simulink model "poco_ref_al_r307"  (Simulink 6.2)
settings: Solver=ode45  StartTime=0.0  StopTime=100000  RelTol=1e-3
libraries: xbsIndex_r3 x1012, xps_library x42, ddc_library x4, adcscope_lib x2, fft_library x2, pfb_library x2, delay_lib x1
(part 3 of 9)

== system poco_ref_al_r307/downshift2 ==
  din : Inport  Port=1  LatchInput=off
  Concat : xbsIndex_r3/Concat  num_inputs=2  explicit_period=off  period=1  dbl_ovrd=off
  Convert1 : xbsIndex_r3/Convert  arith_type="Signed  (2's comp)"  n_bits=18  bin_pt=15  quantization="Round  (unbiased: Even Values)"  overflow=Wrap  latency=2  explicit_period=off  period=1  dbl_ovrd=off  show_param=off  inserted_by_tool=off  pipeline=off
      settings: xl_area=[0, 0, 0, 0, 0, 0, 0]
  Convert2 : xbsIndex_r3/Convert  arith_type="Signed  (2's comp)"  n_bits=18  bin_pt=15  quantization="Round  (unbiased: Even Values)"  overflow=Wrap  latency=2  explicit_period=off  period=1  dbl_ovrd=off  show_param=off  inserted_by_tool=off  pipeline=off
      settings: xl_area=[0, 0, 0, 0, 0, 0, 0]
  Reinterpret : xbsIndex_r3/Reinterpret  force_arith_type=on  arith_type="Signed  (2's comp)"  force_bin_pt=on  bin_pt=17  force_valid=on
  Reinterpret1 : xbsIndex_r3/Reinterpret  force_arith_type=on  arith_type="Signed  (2's comp)"  force_bin_pt=on  bin_pt=17  force_valid=on
  Reinterpret3 : xbsIndex_r3/Reinterpret  force_arith_type=on  arith_type=Unsigned  force_bin_pt=on  bin_pt=0  force_valid=on
  Reinterpret4 : xbsIndex_r3/Reinterpret  force_arith_type=on  arith_type=Unsigned  force_bin_pt=on  bin_pt=0  force_valid=on
  Slice2 : xbsIndex_r3/Slice  mode=Upper Bit Location + Width  nbits=18  bit1=0  base1=MSB of Input  bit0=0  base0=LSB of Input  boolean_output=off  explicit_period=off  period=1  dbl_ovrd=off
  Slice20 : xbsIndex_r3/Slice  mode=Lower Bit Location + Width  nbits=18  bit1=0  base1=MSB of Input  bit0=0  base0=LSB of Input  boolean_output=off  explicit_period=off  period=1  dbl_ovrd=off
  dout : Outport
  wires:
  Convert1/1 -> Reinterpret4/1
  Convert2/1 -> Reinterpret3/1
  Reinterpret1/1 -> Convert1/1
  Reinterpret/1 -> Convert2/1
  Concat/1 -> dout/1
  Reinterpret4/1 -> Concat/2
  Reinterpret3/1 -> Concat/1
  din/1 -> Slice20/1, Slice2/1
  Slice20/1 -> Reinterpret1/1
  Slice2/1 -> Reinterpret/1

== system poco_ref_al_r307/downshift3 ==
  din : Inport  Port=1  LatchInput=off
  Concat : xbsIndex_r3/Concat  num_inputs=2  explicit_period=off  period=1  dbl_ovrd=off
  Convert1 : xbsIndex_r3/Convert  arith_type="Signed  (2's comp)"  n_bits=18  bin_pt=15  quantization="Round  (unbiased: Even Values)"  overflow=Wrap  latency=2  explicit_period=off  period=1  dbl_ovrd=off  show_param=off  inserted_by_tool=off  pipeline=off
      settings: xl_area=[0, 0, 0, 0, 0, 0, 0]
  Convert2 : xbsIndex_r3/Convert  arith_type="Signed  (2's comp)"  n_bits=18  bin_pt=15  quantization="Round  (unbiased: Even Values)"  overflow=Wrap  latency=2  explicit_period=off  period=1  dbl_ovrd=off  show_param=off  inserted_by_tool=off  pipeline=off
      settings: xl_area=[0, 0, 0, 0, 0, 0, 0]
  Reinterpret : xbsIndex_r3/Reinterpret  force_arith_type=on  arith_type="Signed  (2's comp)"  force_bin_pt=on  bin_pt=17  force_valid=on
  Reinterpret1 : xbsIndex_r3/Reinterpret  force_arith_type=on  arith_type="Signed  (2's comp)"  force_bin_pt=on  bin_pt=17  force_valid=on
  Reinterpret3 : xbsIndex_r3/Reinterpret  force_arith_type=on  arith_type=Unsigned  force_bin_pt=on  bin_pt=0  force_valid=on
  Reinterpret4 : xbsIndex_r3/Reinterpret  force_arith_type=on  arith_type=Unsigned  force_bin_pt=on  bin_pt=0  force_valid=on
  Slice2 : xbsIndex_r3/Slice  mode=Upper Bit Location + Width  nbits=18  bit1=0  base1=MSB of Input  bit0=0  base0=LSB of Input  boolean_output=off  explicit_period=off  period=1  dbl_ovrd=off
  Slice20 : xbsIndex_r3/Slice  mode=Lower Bit Location + Width  nbits=18  bit1=0  base1=MSB of Input  bit0=0  base0=LSB of Input  boolean_output=off  explicit_period=off  period=1  dbl_ovrd=off
  dout : Outport
  wires:
  Slice2/1 -> Reinterpret/1
  Slice20/1 -> Reinterpret1/1
  din/1 -> Slice2/1, Slice20/1
  Reinterpret3/1 -> Concat/1
  Reinterpret4/1 -> Concat/2
  Concat/1 -> dout/1
  Reinterpret/1 -> Convert2/1
  Reinterpret1/1 -> Convert1/1
  Convert2/1 -> Reinterpret3/1
  Convert1/1 -> Reinterpret4/1

== system poco_ref_al_r307/eq_ant0 ==
  sync : Inport  Port=1  LatchInput=off
  pol1 : Inport  Port=2  LatchInput=off
  pol2 : Inport  Port=3  LatchInput=off
  scale_pol1 : Inport  Port=4  LatchInput=off
  scale_pol2 : Inport  Port=5  LatchInput=off
  Concat3 : xbsIndex_r3/Concat  num_inputs=2  explicit_period=off  period=1  dbl_ovrd=off
  Delay1 : xbsIndex_r3/Delay  latency=1  reg_retiming=off  explicit_period=off  period=1  en=off  accept_only_valid=off  init_zero=on  dbl_ovrd=off  show_param=off
      settings: xl_area=[0, 0, 0, 0, 0, 0, 0]
  Delay11 : xbsIndex_r3/Delay  latency=1  reg_retiming=off  explicit_period=off  period=1  en=off  accept_only_valid=off  init_zero=on  dbl_ovrd=off  show_param=off
      settings: xl_area=[0, 0, 0, 0, 0, 0, 0]
  Delay4 : xbsIndex_r3/Delay  latency=5  reg_retiming=off  explicit_period=off  period=1  en=off  accept_only_valid=off  init_zero=on  dbl_ovrd=off  show_param=off
      settings: xl_area=[0, 0, 0, 0, 0, 0, 0]
  Logical1 : xbsIndex_r3/Logical  logical_function=OR  inputs=2  precision=Full  arith_type=Unsigned  n_bits=8  bin_pt=2  align_bp=on  latency=1  explicit_period=off  period=1  en=off  dbl_ovrd=off  show_param=off
      settings: xl_area=[0, 0, 0, 0, 0, 0, 0]
  round1 : Subsystem
  round2 : Subsystem
  dout : Outport
  sync_out : Outport  Port=2
  clip : Outport  Port=3
  wires:
  sync/1 -> Delay4/1
  round1/1(dout) -> Concat3/1
  round2/1(dout) -> Concat3/2
  Delay11/1 -> round1/1(din)
  Delay1/1 -> round2/1(din)
  pol1/1 -> Delay11/1
  pol2/1 -> Delay1/1
  Concat3/1 -> dout/1
  Delay4/1 -> sync_out/1
  round1/2(clip) -> Logical1/1
  round2/2(clip) -> Logical1/2
  Logical1/1 -> clip/1
  scale_pol1/1 -> round1/2(scale)
  scale_pol2/1 -> round2/2(scale)

== system poco_ref_al_r307/eq_ant1 ==
  sync : Inport  Port=1  LatchInput=off
  pol1 : Inport  Port=2  LatchInput=off
  pol2 : Inport  Port=3  LatchInput=off
  scale_pol1 : Inport  Port=4  LatchInput=off
  scale_pol2 : Inport  Port=5  LatchInput=off
  Concat3 : xbsIndex_r3/Concat  num_inputs=2  explicit_period=off  period=1  dbl_ovrd=off
  Delay1 : xbsIndex_r3/Delay  latency=1  reg_retiming=off  explicit_period=off  period=1  en=off  accept_only_valid=off  init_zero=on  dbl_ovrd=off  show_param=off
      settings: xl_area=[0, 0, 0, 0, 0, 0, 0]
  Delay11 : xbsIndex_r3/Delay  latency=1  reg_retiming=off  explicit_period=off  period=1  en=off  accept_only_valid=off  init_zero=on  dbl_ovrd=off  show_param=off
      settings: xl_area=[0, 0, 0, 0, 0, 0, 0]
  Delay4 : xbsIndex_r3/Delay  latency=5  reg_retiming=off  explicit_period=off  period=1  en=off  accept_only_valid=off  init_zero=on  dbl_ovrd=off  show_param=off
      settings: xl_area=[0, 0, 0, 0, 0, 0, 0]
  Logical1 : xbsIndex_r3/Logical  logical_function=OR  inputs=2  precision=Full  arith_type=Unsigned  n_bits=8  bin_pt=2  align_bp=on  latency=1  explicit_period=off  period=1  en=off  dbl_ovrd=off  show_param=off
      settings: xl_area=[0, 0, 0, 0, 0, 0, 0]
  round1 : Subsystem
  round2 : Subsystem
  dout : Outport
  sync_out : Outport  Port=2
  clip : Outport  Port=3
  wires:
  scale_pol2/1 -> round2/2(scale)
  scale_pol1/1 -> round1/2(scale)
  Logical1/1 -> clip/1
  round2/2(clip) -> Logical1/2
  round1/2(clip) -> Logical1/1
  Delay4/1 -> sync_out/1
  Concat3/1 -> dout/1
  pol2/1 -> Delay1/1
  pol1/1 -> Delay11/1
  Delay1/1 -> round2/1(din)
  Delay11/1 -> round1/1(din)
  round2/1(dout) -> Concat3/2
  round1/1(dout) -> Concat3/1
  sync/1 -> Delay4/1

== system poco_ref_al_r307/eq_prog ==
  sync : Inport  Port=1  LatchInput=off
  data_in : Inport  Port=2  LatchInput=off
  addr_in : Inport  Port=3  LatchInput=off
  valid_in : Inport  Port=4  LatchInput=off
  Constant : xbsIndex_r3/Constant  const=addr_offset  equ=P=C  arith_type=Unsigned  n_bits=32-addr_width  bin_pt=0  opselect=C  inp2=PCIN>>17  opr=+  inp1=P  carry=CIN  iostate=0  explicit_period=on  period=1  dbl_ovrd=off
  Constant5 : xbsIndex_r3/Constant  const=0  equ=P=C  arith_type=Unsigned  n_bits=16  bin_pt=3  opselect=C  inp2=PCIN>>17  opr=+  inp1=P  carry=CIN  iostate=0  explicit_period=on  period=1  dbl_ovrd=off
  Constant6 : xbsIndex_r3/Constant  const=0  equ=P=C  arith_type=Boolean  n_bits=1  bin_pt=0  opselect=C  inp2=PCIN>>17  opr=+  inp1=P  carry=CIN  iostate=0  explicit_period=on  period=1  dbl_ovrd=off
  Counter2 : xbsIndex_r3/Counter  cnt_type=Free Running  n_bits=chan_bits  bin_pt=0  arith_type=Unsigned  start_count=0  cnt_to=Inf  cnt_by_val=1  operation=Up  explicit_period=off  period=1  load_pin=off  rst=on  en=off  dbl_ovrd=off  show_param=off  use_rpm=on  gen_core=off
      settings: xl_area=[0, 0, 0, 0, 0, 0, 0]
  Dual Port RAM : xbsIndex_r3/Dual Port RAM  depth=n_chans  initVector=ones(1,n_chans)*1000  write_mode_A=Read After Write  write_mode_B=Read After Write  latency=1  mem_collision=off  init_zero=on  explicit_period=off  period=1  dbl_ovrd=off  rst_a=off  init_a=0  rst_b=off  init_b=0  show_param=off  distributed_mem=off  use_rpm=off  gen_core=off
      settings: xl_area=[0, 0, 0, 0, 0, 0, 0]
  Logical : xbsIndex_r3/Logical  logical_function=AND  inputs=2  precision=Full  arith_type=Unsigned  n_bits=8  bin_pt=2  align_bp=on  latency=0  explicit_period=off  period=1  en=off  dbl_ovrd=off  show_param=off
      settings: xl_area=[0, 0, 0, 0, 0, 0, 0]
  Register1 : xbsIndex_r3/Register  init=0  reg_only_valid=off  explicit_period=on  period=1  rst=off  en=off  out_en=off  dbl_ovrd=off  show_param=off
      settings: xl_area=[0, 0, 0, 0, 0, 0, 0]
  Register2 : xbsIndex_r3/Register  init=0  reg_only_valid=off  explicit_period=on  period=1  rst=off  en=off  out_en=off  dbl_ovrd=off  show_param=off
      settings: xl_area=[0, 0, 0, 0, 0, 0, 0]
  Register3 : xbsIndex_r3/Register  init=0  reg_only_valid=off  explicit_period=on  period=1  rst=off  en=off  out_en=off  dbl_ovrd=off  show_param=off
      settings: xl_area=[0, 0, 0, 0, 0, 0, 0]
  Reinterpret1 : xbsIndex_r3/Reinterpret  force_arith_type=on  arith_type=Unsigned  force_bin_pt=on  bin_pt=3  force_valid=on
  Relational : xbsIndex_r3/Relational  mode=a=b  latency=1  explicit_period=on  period=1  en=off  dbl_ovrd=off  show_param=off
      settings: xl_area=[0, 0, 0, 0, 0, 0, 0]
  Slice22 : xbsIndex_r3/Slice  mode=Lower Bit Location + Width  nbits=32-addr_width  bit1=0  base1=MSB of Input  bit0=addr_width  base0=LSB of Input  boolean_output=off  explicit_period=off  period=1  dbl_ovrd=off
  Slice9 : xbsIndex_r3/Slice  mode=Lower Bit Location + Width  nbits=addr_width  bit1=0  base1=MSB of Input  bit0=0  base0=LSB of Input  boolean_output=off  explicit_period=off  period=1  dbl_ovrd=off
  scale : Outport
  wires:
  addr_in/1 -> Slice9/1, Slice22/1
  Slice22/1 -> Relational/1
  Constant/1 -> Relational/2
  Relational/1 -> Logical/1
  valid_in/1 -> Register3/1
  Logical/1 -> Dual Port RAM/6
  Slice9/1 -> Register2/1
  data_in/1 -> Register1/1
  Register1/1 -> Reinterpret1/1
  Register2/1 -> Dual Port RAM/4
  Register3/1 -> Logical/2
  Counter2/1 -> Dual Port RAM/1
  Constant5/1 -> Dual Port RAM/2
  Constant6/1 -> Dual Port RAM/3
  Reinterpret1/1 -> Dual Port RAM/5
  sync/1 -> Counter2/1
  Dual Port RAM/1 -> scale/1

== system poco_ref_al_r307/pulse_ext1 ==
  in : Inport  Port=1  LatchInput=off
  Constant5 : xbsIndex_r3/Constant  const=pulse_len  equ=P=C  arith_type=Unsigned  n_bits=bits  bin_pt=0  opselect=C  inp2=PCIN>>17  opr=+  inp1=P  carry=CIN  iostate=0  explicit_period=off  period=1  dbl_ovrd=off
  Counter3 : xbsIndex_r3/Counter  cnt_type=Free Running  n_bits=bits  bin_pt=0  arith_type=Unsigned  start_count=0  cnt_to=1023  cnt_by_val=1  operation=Up  explicit_period=on  period=1  load_pin=off  rst=on  en=on  dbl_ovrd=off  show_param=off  use_rpm=on  gen_core=off
      settings: xl_area=[0, 0, 0, 0, 0, 0, 0]
  Relational5 : xbsIndex_r3/Relational  mode=a!=b  latency=0  explicit_period=off  period=1  en=off  dbl_ovrd=off  show_param=off
      settings: xl_area=[0, 0, 0, 0, 0, 0, 0]
  posedge : Subsystem  Tag=Rising Edge Detector
  out : Outport
  wires:
  posedge/1(Out) -> Counter3/1
  in/1 -> posedge/1(In)
  Relational5/1 -> out/1, Counter3/2
  Constant5/1 -> Relational5/2
  Counter3/1 -> Relational5/1

== system poco_ref_al_r307/pulse_ext2 ==
  in : Inport  Port=1  LatchInput=off
  Constant5 : xbsIndex_r3/Constant  const=pulse_len  equ=P=C  arith_type=Unsigned  n_bits=bits  bin_pt=0  opselect=C  inp2=PCIN>>17  opr=+  inp1=P  carry=CIN  iostate=0  explicit_period=off  period=1  dbl_ovrd=off
  Counter3 : xbsIndex_r3/Counter  cnt_type=Free Running  n_bits=bits  bin_pt=0  arith_type=Unsigned  start_count=0  cnt_to=1023  cnt_by_val=1  operation=Up  explicit_period=on  period=1  load_pin=off  rst=on  en=on  dbl_ovrd=off  show_param=off  use_rpm=on  gen_core=off
      settings: xl_area=[0, 0, 0, 0, 0, 0, 0]
  Relational5 : xbsIndex_r3/Relational  mode=a!=b  latency=0  explicit_period=off  period=1  en=off  dbl_ovrd=off  show_param=off
      settings: xl_area=[0, 0, 0, 0, 0, 0, 0]
  posedge : Subsystem  Tag=Rising Edge Detector
  out : Outport
  wires:
  Counter3/1 -> Relational5/1
  Constant5/1 -> Relational5/2
  Relational5/1 -> Counter3/2, out/1
  in/1 -> posedge/1(In)
  posedge/1(Out) -> Counter3/1

== system poco_ref_al_r307/pulse_ext3 ==
  in : Inport  Port=1  LatchInput=off
  Constant5 : xbsIndex_r3/Constant  const=pulse_len  equ=P=C  arith_type=Unsigned  n_bits=bits  bin_pt=0  opselect=C  inp2=PCIN>>17  opr=+  inp1=P  carry=CIN  iostate=0  explicit_period=off  period=1  dbl_ovrd=off
  Counter3 : xbsIndex_r3/Counter  cnt_type=Free Running  n_bits=bits  bin_pt=0  arith_type=Unsigned  start_count=0  cnt_to=1023  cnt_by_val=1  operation=Up  explicit_period=on  period=1  load_pin=off  rst=on  en=on  dbl_ovrd=off  show_param=off  use_rpm=on  gen_core=off
      settings: xl_area=[0, 0, 0, 0, 0, 0, 0]
  Relational5 : xbsIndex_r3/Relational  mode=a!=b  latency=0  explicit_period=off  period=1  en=off  dbl_ovrd=off  show_param=off
      settings: xl_area=[0, 0, 0, 0, 0, 0, 0]
  posedge : Subsystem  Tag=Rising Edge Detector
  out : Outport
  wires:
  Counter3/1 -> Relational5/1
  Constant5/1 -> Relational5/2
  Relational5/1 -> Counter3/2, out/1
  in/1 -> posedge/1(In)
  posedge/1(Out) -> Counter3/1

== system poco_ref_al_r307/pulse_ext4 ==
  in : Inport  Port=1  LatchInput=off
  Constant5 : xbsIndex_r3/Constant  const=pulse_len  equ=P=C  arith_type=Unsigned  n_bits=bits  bin_pt=0  opselect=C  inp2=PCIN>>17  opr=+  inp1=P  carry=CIN  iostate=0  explicit_period=off  period=1  dbl_ovrd=off
  Counter3 : xbsIndex_r3/Counter  cnt_type=Free Running  n_bits=bits  bin_pt=0  arith_type=Unsigned  start_count=0  cnt_to=1023  cnt_by_val=1  operation=Up  explicit_period=on  period=1  load_pin=off  rst=on  en=on  dbl_ovrd=off  show_param=off  use_rpm=on  gen_core=off
      settings: xl_area=[0, 0, 0, 0, 0, 0, 0]
  Relational5 : xbsIndex_r3/Relational  mode=a!=b  latency=0  explicit_period=off  period=1  en=off  dbl_ovrd=off  show_param=off
      settings: xl_area=[0, 0, 0, 0, 0, 0, 0]
  posedge : Subsystem  Tag=Rising Edge Detector
  out : Outport
  wires:
  Counter3/1 -> Relational5/1
  Constant5/1 -> Relational5/2
  Relational5/1 -> Counter3/2, out/1
  in/1 -> posedge/1(In)
  posedge/1(Out) -> Counter3/1

== system poco_ref_al_r307/pulse_ext5 ==
  in : Inport  Port=1  LatchInput=off
  Constant5 : xbsIndex_r3/Constant  const=pulse_len  equ=P=C  arith_type=Unsigned  n_bits=bits  bin_pt=0  opselect=C  inp2=PCIN>>17  opr=+  inp1=P  carry=CIN  iostate=0  explicit_period=off  period=1  dbl_ovrd=off
  Counter3 : xbsIndex_r3/Counter  cnt_type=Free Running  n_bits=bits  bin_pt=0  arith_type=Unsigned  start_count=0  cnt_to=1023  cnt_by_val=1  operation=Up  explicit_period=on  period=1  load_pin=off  rst=on  en=on  dbl_ovrd=off  show_param=off  use_rpm=on  gen_core=off
      settings: xl_area=[0, 0, 0, 0, 0, 0, 0]
  Relational5 : xbsIndex_r3/Relational  mode=a!=b  latency=0  explicit_period=off  period=1  en=off  dbl_ovrd=off  show_param=off
      settings: xl_area=[0, 0, 0, 0, 0, 0, 0]
  posedge : Subsystem  Tag=Rising Edge Detector
  out : Outport
  wires:
  posedge/1(Out) -> Counter3/1
  in/1 -> posedge/1(In)
  Relational5/1 -> out/1, Counter3/2
  Constant5/1 -> Relational5/2
  Counter3/1 -> Relational5/1

== system poco_ref_al_r307/pulse_ext6 ==
  in : Inport  Port=1  LatchInput=off
  Constant5 : xbsIndex_r3/Constant  const=pulse_len  equ=P=C  arith_type=Unsigned  n_bits=bits  bin_pt=0  opselect=C  inp2=PCIN>>17  opr=+  inp1=P  carry=CIN  iostate=0  explicit_period=off  period=1  dbl_ovrd=off
  Counter3 : xbsIndex_r3/Counter  cnt_type=Free Running  n_bits=bits  bin_pt=0  arith_type=Unsigned  start_count=0  cnt_to=1023  cnt_by_val=1  operation=Up  explicit_period=on  period=1  load_pin=off  rst=on  en=on  dbl_ovrd=off  show_param=off  use_rpm=on  gen_core=off
      settings: xl_area=[0, 0, 0, 0, 0, 0, 0]
  Relational5 : xbsIndex_r3/Relational  mode=a!=b  latency=0  explicit_period=off  period=1  en=off  dbl_ovrd=off  show_param=off
      settings: xl_area=[0, 0, 0, 0, 0, 0, 0]
  posedge : Subsystem  Tag=Rising Edge Detector
  out : Outport
  wires:
  posedge/1(Out) -> Counter3/1
  in/1 -> posedge/1(In)
  Relational5/1 -> out/1, Counter3/2
  Constant5/1 -> Relational5/2
  Counter3/1 -> Relational5/1

== system poco_ref_al_r307/pulse_ext7 ==
  in : Inport  Port=1  LatchInput=off
  Constant5 : xbsIndex_r3/Constant  const=pulse_len  equ=P=C  arith_type=Unsigned  n_bits=bits  bin_pt=0  opselect=C  inp2=PCIN>>17  opr=+  inp1=P  carry=CIN  iostate=0  explicit_period=off  period=1  dbl_ovrd=off
  Counter3 : xbsIndex_r3/Counter  cnt_type=Free Running  n_bits=bits  bin_pt=0  arith_type=Unsigned  start_count=0  cnt_to=1023  cnt_by_val=1  operation=Up  explicit_period=on  period=1  load_pin=off  rst=on  en=on  dbl_ovrd=off  show_param=off  use_rpm=on  gen_core=off
      settings: xl_area=[0, 0, 0, 0, 0, 0, 0]
  Relational5 : xbsIndex_r3/Relational  mode=a!=b  latency=0  explicit_period=off  period=1  en=off  dbl_ovrd=off  show_param=off
      settings: xl_area=[0, 0, 0, 0, 0, 0, 0]
  posedge : Subsystem  Tag=Rising Edge Detector
  out : Outport
  wires:
  posedge/1(Out) -> Counter3/1
  in/1 -> posedge/1(In)
  Relational5/1 -> out/1, Counter3/2
  Constant5/1 -> Relational5/2
  Counter3/1 -> Relational5/1

== system poco_ref_al_r307/sync_gen ==
  note: sync_delay makes sure mrst
      | gets transmitted
      | on a correctly aligned sync
  rst : Inport  Port=1  LatchInput=off
  arm : Inport  Port=2  LatchInput=off
  Constant10 : xbsIndex_r3/Constant  const=1  equ=P=C  arith_type=Boolean  n_bits=1  bin_pt=0  opselect=C  inp2=PCIN>>17  opr=+  inp1=P  carry=CIN  iostate=0  explicit_period=on  period=1  dbl_ovrd=off
  Counter : xbsIndex_r3/Counter  cnt_type=Free Running  n_bits=sync_bits+1  bin_pt=0  arith_type=Unsigned  start_count=0  cnt_to=Inf  cnt_by_val=1  operation=Up  explicit_period=off  period=1  load_pin=off  rst=on  en=off  dbl_ovrd=off  show_param=off  use_rpm=on  gen_core=off
      settings: xl_area=[0, 0, 0, 0, 0, 0, 0]
  Inverter : xbsIndex_r3/Inverter  latency=2  explicit_period=off  period=1  en=off  dbl_ovrd=off  show_param=off
      settings: xl_area=[0, 0, 0, 0, 0, 0, 0]
  Register : xbsIndex_r3/Register  init=0  reg_only_valid=off  explicit_period=off  period=1  rst=on  en=on  out_en=off  dbl_ovrd=off  show_param=off
      settings: xl_area=[0, 0, 0, 0, 0, 0, 0]
  Slice8 : xbsIndex_r3/Slice  mode=Upper Bit Location + Width  nbits=1  bit1=0  base1=MSB of Input  bit0=19  base0=LSB of Input  boolean_output=on  explicit_period=off  period=1  dbl_ovrd=off
  edge : Subsystem
  posedge1 : Subsystem  Tag=Rising Edge Detector
  posedge2 : Subsystem  Tag=Rising Edge Detector
  sync_delay : delay_lib/sync_delay  DelayLen=2^sync_bits
      link override Constant: equ=P=C
      link override Constant1: equ=P=C
      link override Constant2: equ=P=C
      link override Constant3: equ=P=C
  sync : Outport
  mrst : Outport  Port=2
  armed : Outport  Port=3
  wires:
  Counter/1 -> Slice8/1
  posedge1/1(Out) -> Counter/1, sync_delay/1
  Register/1 -> posedge1/1(In), Inverter/1
  Constant10/1 -> Register/1
  posedge2/1(Out) -> Register/2
  arm/1 -> posedge2/1(In)
  rst/1 -> Register/3
  sync_delay/1 -> mrst/1
  Slice8/1 -> edge/1(in)
  edge/1(out) -> sync/1
  Inverter/1 -> armed/1

== system poco_ref_al_r307/acc_cntrl/posedge1 ==
  In : Inport  Port=1  LatchInput=off
  Delay : xbsIndex_r3/Delay  latency=1  reg_retiming=off  explicit_period=off  period=1  en=off  accept_only_valid=off  init_zero=on  dbl_ovrd=off  show_param=off
      settings: xl_area=[0, 0, 0, 0, 0, 0, 0]
  Inverter : xbsIndex_r3/Inverter  latency=0  explicit_period=off  period=1  en=off  dbl_ovrd=off  show_param=off
      settings: xl_area=[0, 0, 0, 0, 0, 0, 0]
  Logical : xbsIndex_r3/Logical  logical_function=AND  inputs=2  precision=Full  arith_type=Unsigned  n_bits=8  bin_pt=2  align_bp=on  latency=0  explicit_period=off  period=1  en=off  dbl_ovrd=off  show_param=off
      settings: xl_area=[0, 0, 0, 0, 0, 0, 0]
  Out : Outport
  wires:
  Logical/1 -> Out/1
  In/1 -> Logical/2, Delay/1
  Inverter/1 -> Logical/1
  Delay/1 -> Inverter/1

== system poco_ref_al_r307/acc_cntrl/posedge2 ==
  In : Inport  Port=1  LatchInput=off
  Delay : xbsIndex_r3/Delay  latency=1  reg_retiming=off  explicit_period=off  period=1  en=off  accept_only_valid=off  init_zero=on  dbl_ovrd=off  show_param=off
      settings: xl_area=[0, 0, 0, 0, 0, 0, 0]
  Inverter : xbsIndex_r3/Inverter  latency=0  explicit_period=off  period=1  en=off  dbl_ovrd=off  show_param=off
      settings: xl_area=[0, 0, 0, 0, 0, 0, 0]
  Logical : xbsIndex_r3/Logical  logical_function=AND  inputs=2  precision=Full  arith_type=Unsigned  n_bits=8  bin_pt=2  align_bp=on  latency=0  explicit_period=off  period=1  en=off  dbl_ovrd=off  show_param=off
      settings: xl_area=[0, 0, 0, 0, 0, 0, 0]
  Out : Outport
  wires:
  Delay/1 -> Inverter/1
  Inverter/1 -> Logical/1
  In/1 -> Delay/1, Logical/2
  Logical/1 -> Out/1

== system poco_ref_al_r307/calc_adc_sum_sq1/decat4 ==
  In1 : Inport  Port=1  LatchInput=off
  Reinterpret{1..4} (4 alike) : xbsIndex_r3/Reinterpret  force_arith_type=on  arith_type="Signed  (2's comp)"  force_bin_pt=on  bin_pt=7  force_valid=on
  Slice15 : xbsIndex_r3/Slice  mode=Lower Bit Location + Width  nbits=8  bit1=0  base1=MSB of Input  bit0=8  base0=LSB of Input  boolean_output=off  explicit_period=off  period=1  dbl_ovrd=off
  Slice16 : xbsIndex_r3/Slice  mode=Lower Bit Location + Width  nbits=8  bit1=0  base1=MSB of Input  bit0=16  base0=LSB of Input  boolean_output=off  explicit_period=off  period=1  dbl_ovrd=off
  Slice17 : xbsIndex_r3/Slice  mode=Lower Bit Location + Width  nbits=8  bit1=0  base1=MSB of Input  bit0=24  base0=LSB of Input  boolean_output=off  explicit_period=off  period=1  dbl_ovrd=off
  Slice9 : xbsIndex_r3/Slice  mode=Lower Bit Location + Width  nbits=8  bit1=0  base1=MSB of Input  bit0=0  base0=LSB of Input  boolean_output=off  explicit_period=off  period=1  dbl_ovrd=off
  Out1 : Outport
  Out2 : Outport  Port=2
  Out3 : Outport  Port=3
  Out4 : Outport  Port=4
  wires:
  Reinterpret4/1 -> Out4/1
  Reinterpret3/1 -> Out3/1
  Reinterpret1/1 -> Out2/1
  Reinterpret2/1 -> Out1/1
  Slice9/1 -> Reinterpret4/1
  Slice15/1 -> Reinterpret3/1
  Slice16/1 -> Reinterpret1/1
  Slice17/1 -> Reinterpret2/1
  In1/1 -> Slice15/1, Slice9/1, Slice16/1, Slice17/1

== system poco_ref_al_r307/calc_adc_sum_sq2/decat4 ==
  In1 : Inport  Port=1  LatchInput=off
  Reinterpret{1..4} (4 alike) : xbsIndex_r3/Reinterpret  force_arith_type=on  arith_type="Signed  (2's comp)"  force_bin_pt=on  bin_pt=7  force_valid=on
  Slice15 : xbsIndex_r3/Slice  mode=Lower Bit Location + Width  nbits=8  bit1=0  base1=MSB of Input  bit0=8  base0=LSB of Input  boolean_output=off  explicit_period=off  period=1  dbl_ovrd=off
  Slice16 : xbsIndex_r3/Slice  mode=Lower Bit Location + Width  nbits=8  bit1=0  base1=MSB of Input  bit0=16  base0=LSB of Input  boolean_output=off  explicit_period=off  period=1  dbl_ovrd=off
  Slice17 : xbsIndex_r3/Slice  mode=Lower Bit Location + Width  nbits=8  bit1=0  base1=MSB of Input  bit0=24  base0=LSB of Input  boolean_output=off  explicit_period=off  period=1  dbl_ovrd=off
  Slice9 : xbsIndex_r3/Slice  mode=Lower Bit Location + Width  nbits=8  bit1=0  base1=MSB of Input  bit0=0  base0=LSB of Input  boolean_output=off  explicit_period=off  period=1  dbl_ovrd=off
  Out1 : Outport
  Out2 : Outport  Port=2
  Out3 : Outport  Port=3
  Out4 : Outport  Port=4
  wires:
  Reinterpret4/1 -> Out4/1
  Reinterpret3/1 -> Out3/1
  Reinterpret1/1 -> Out2/1
  Reinterpret2/1 -> Out1/1
  Slice9/1 -> Reinterpret4/1
  Slice15/1 -> Reinterpret3/1
  Slice16/1 -> Reinterpret1/1
  Slice17/1 -> Reinterpret2/1
  In1/1 -> Slice15/1, Slice9/1, Slice16/1, Slice17/1

== system poco_ref_al_r307/calc_adc_sum_sq3/decat4 ==
  In1 : Inport  Port=1  LatchInput=off
  Reinterpret{1..4} (4 alike) : xbsIndex_r3/Reinterpret  force_arith_type=on  arith_type="Signed  (2's comp)"  force_bin_pt=on  bin_pt=7  force_valid=on
  Slice15 : xbsIndex_r3/Slice  mode=Lower Bit Location + Width  nbits=8  bit1=0  base1=MSB of Input  bit0=8  base0=LSB of Input  boolean_output=off  explicit_period=off  period=1  dbl_ovrd=off
  Slice16 : xbsIndex_r3/Slice  mode=Lower Bit Location + Width  nbits=8  bit1=0  base1=MSB of Input  bit0=16  base0=LSB of Input  boolean_output=off  explicit_period=off  period=1  dbl_ovrd=off
  Slice17 : xbsIndex_r3/Slice  mode=Lower Bit Location + Width  nbits=8  bit1=0  base1=MSB of Input  bit0=24  base0=LSB of Input  boolean_output=off  explicit_period=off  period=1  dbl_ovrd=off
  Slice9 : xbsIndex_r3/Slice  mode=Lower Bit Location + Width  nbits=8  bit1=0  base1=MSB of Input  bit0=0  base0=LSB of Input  boolean_output=off  explicit_period=off  period=1  dbl_ovrd=off
  Out1 : Outport
  Out2 : Outport  Port=2
  Out3 : Outport  Port=3
  Out4 : Outport  Port=4
  wires:
  Reinterpret4/1 -> Out4/1
  Reinterpret3/1 -> Out3/1
  Reinterpret1/1 -> Out2/1
  Reinterpret2/1 -> Out1/1
  Slice9/1 -> Reinterpret4/1
  Slice15/1 -> Reinterpret3/1
  Slice16/1 -> Reinterpret1/1
  Slice17/1 -> Reinterpret2/1
  In1/1 -> Slice15/1, Slice9/1, Slice16/1, Slice17/1

== system poco_ref_al_r307/calc_adc_sum_sq4/decat4 ==
  In1 : Inport  Port=1  LatchInput=off
  Reinterpret{1..4} (4 alike) : xbsIndex_r3/Reinterpret  force_arith_type=on  arith_type="Signed  (2's comp)"  force_bin_pt=on  bin_pt=7  force_valid=on
  Slice15 : xbsIndex_r3/Slice  mode=Lower Bit Location + Width  nbits=8  bit1=0  base1=MSB of Input  bit0=8  base0=LSB of Input  boolean_output=off  explicit_period=off  period=1  dbl_ovrd=off
  Slice16 : xbsIndex_r3/Slice  mode=Lower Bit Location + Width  nbits=8  bit1=0  base1=MSB of Input  bit0=16  base0=LSB of Input  boolean_output=off  explicit_period=off  period=1  dbl_ovrd=off
  Slice17 : xbsIndex_r3/Slice  mode=Lower Bit Location + Width  nbits=8  bit1=0  base1=MSB of Input  bit0=24  base0=LSB of Input  boolean_output=off  explicit_period=off  period=1  dbl_ovrd=off
  Slice9 : xbsIndex_r3/Slice  mode=Lower Bit Location + Width  nbits=8  bit1=0  base1=MSB of Input  bit0=0  base0=LSB of Input  boolean_output=off  explicit_period=off  period=1  dbl_ovrd=off
  Out1 : Outport
  Out2 : Outport  Port=2
  Out3 : Outport  Port=3
  Out4 : Outport  Port=4
  wires:
  Reinterpret4/1 -> Out4/1
  Reinterpret3/1 -> Out3/1
  Reinterpret1/1 -> Out2/1
  Reinterpret2/1 -> Out1/1
  Slice9/1 -> Reinterpret4/1
  Slice15/1 -> Reinterpret3/1
  Slice16/1 -> Reinterpret1/1
  Slice17/1 -> Reinterpret2/1
  In1/1 -> Slice15/1, Slice9/1, Slice16/1, Slice17/1

== system poco_ref_al_r307/delay_wideband_prog0/barrel_switcher ==
  sel : Inport  Port=1  LatchInput=off
  sync_in : Inport  Port=2  LatchInput=off
  In1 : Inport  Port=3  LatchInput=off
  In2 : Inport  Port=4  LatchInput=off
  In3 : Inport  Port=5  LatchInput=off
  In4 : Inport  Port=6  LatchInput=off
  Delay1 : xbsIndex_r3/Delay  latency=1  reg_retiming=off  explicit_period=off  period=1  en=off  accept_only_valid=off  init_zero=on  dbl_ovrd=off  show_param=off
      settings: xl_area=[0, 0, 0, 0, 0, 0, 0]
  Delay_sync : xbsIndex_r3/Delay  latency=2  reg_retiming=off  explicit_period=off  period=1  en=off  accept_only_valid=off  init_zero=on  dbl_ovrd=off  show_param=off
      settings: xl_area=[0, 0, 0, 0, 0, 0, 0]
  Mux{11..12,21..22,31..32,41..42} (8 alike) : xbsIndex_r3/Mux  inputs=2  precision=Full  arith_type="Signed  (2's comp)"  n_bits=8  bin_pt=2  quantization=Truncate  overflow=Wrap  latency=1  explicit_period=off  period=1  en=off  dbl_ovrd=off  show_param=off  mux_type=off  use_rpm=off  gen_core=off
      settings: xl_area=[0, 0, 0, 0, 0, 0, 0]
  Slice1 : xbsIndex_r3/Slice  mode=Upper Bit Location + Width  nbits=1  bit1=-0  base1=MSB of Input  bit0=0  base0=LSB of Input  boolean_output=off  explicit_period=off  period=1  dbl_ovrd=off
  Slice2 : xbsIndex_r3/Slice  mode=Upper Bit Location + Width  nbits=1  bit1=-1  base1=MSB of Input  bit0=0  base0=LSB of Input  boolean_output=off  explicit_period=off  period=1  dbl_ovrd=off
  sync_out : Outport
  Out1 : Outport  Port=2
  Out2 : Outport  Port=3
  Out3 : Outport  Port=4
  Out4 : Outport  Port=5
  wires:
  sync_in/1 -> Delay_sync/1
  Delay_sync/1 -> sync_out/1
  sel/1 -> Slice1/1, Delay1/1
  Delay1/1 -> Slice2/1
  Slice1/1 -> Mux11/1, Mux21/1, Mux31/1, Mux41/1
  Slice2/1 -> Mux12/1, Mux22/1, Mux32/1, Mux42/1
  In1/1 -> Mux11/2, Mux31/3
  Mux12/1 -> Out1/1
  In2/1 -> Mux21/2, Mux41/3
  Mux22/1 -> Out2/1
  In3/1 -> Mux31/2, Mux11/3
  Mux32/1 -> Out3/1
  In4/1 -> Mux41/2, Mux21/3
  Mux42/1 -> Out4/1
  Mux11/1 -> Mux12/2, Mux42/3
  Mux21/1 -> Mux22/2, Mux12/3
  Mux31/1 -> Mux32/2, Mux22/3
  Mux41/1 -> Mux42/2, Mux32/3

== system poco_ref_al_r307/delay_wideband_prog0/delay_dp ==
  din : Inport  Port=1  LatchInput=off
  delay : Inport  Port=2  LatchInput=off
  AddSub : xbsIndex_r3/AddSub  mode=Subtraction  precision=User Defined  arith_type=Unsigned  n_bits=11  bin_pt=0  quantization=Truncate  overflow=Wrap  latency=1  explicit_period=off  period=1  use_carryin=off  use_carryout=off  en=off  dbl_ovrd=off  show_param=off  use_core=on  pipeline=off  use_rpm=on  gen_core=off
      settings: xl_area=[0, 0, 0, 0, 0, 0, 0]
  Constant2 : xbsIndex_r3/Constant  const=1  equ=P=C  arith_type=Boolean  n_bits=1  bin_pt=0  opselect=C  inp2=PCIN>>17  opr=+  inp1=P  carry=CIN  iostate=0  explicit_period=on  period=1  dbl_ovrd=off
  Constant4 : xbsIndex_r3/Constant  const=0  equ=P=C  arith_type=Boolean  n_bits=1  bin_pt=0  opselect=C  inp2=PCIN>>17  opr=+  inp1=P  carry=CIN  iostate=0  explicit_period=on  period=1  dbl_ovrd=off
  Dual Port RAM : S-Function  AncestorBlock=xbsIndex_r3/Dual Port RAM  FunctionName=xldpram  Parameters=sfcn_mwsv__  mask(Xilinx Dual Port Random Access Memory){depth=2048, initVector=0, write_mode_A=Read After Write, write_mode_B=Read After Write, latency=4, mem_collision=off, init_zero=on, explicit_period=off, period=1, dbl_ovrd=off, rst_a=off, init_a=0, rst_b=off, init_b=0, show_param=off, distributed_mem=off, use_rpm=off, gen_core=off, xl_area=[0, 0, 0, 0, 0, 0, 0], xl_use_area=off}
      mask prompts: initVector "Initial Value Vector"; write_mode_A "Write Mode:  Port A"; write_mode_B "Write Mode:  Port B"; mem_collision "Provide Output Valid Port"; init_zero "Zero Initial Output  (otherwise NaN)"; explicit_period "Use Explicit Sample Period"; period "Sample Period  (use -1 to inherit first known input period)"; dbl_ovrd "Override with Doubles"; rst_a "Provide Reset Port for Port A Output Register"; init_a "Initial Value for Port A Output Register"; rst_b "Provide Reset Port for Port B Output Register"; init_b "Initial Value for Port B Output Register"; show_param "---------------------- Show Implementation Parameters -----------------------------------------------------------------------------------"; distributed_mem "Use Distributed Memory (instead of block RAM)"; use_rpm "Use Placement Information for Core"; gen_core "Generate Core"; xl_area "FPGA Area [Slices, FFs, BRAMs, LUTs, IOBs, Emb. Mults, TBUFs]"; xl_use_area "Use Area Above For Estimation"
      mask help: Dual port random access memory (RAM). Independent address, data and write enable ports allow shared access to a single memory space. Dual ports enable simultaneous access to the memory space at different sample rates using multiple data widths.
      mask init:
      | [designRoot, family, part, speed, package, simulinkPeriod, sysclkPeriod, dbl_ovrd, trimVbit] = xlSysgenSettings(gcb,1,1);
      | if isempty(family)
      | 	family = 'Virtex2';
      | end;
      | dbl_ovrdStr = '';
      | [bg,fg] = xlcmap('XBlock',dbl_ovrd);
      | iPos = get_param(gcb,'Position');
      | iWidth=iPos(3)-iPos(1); iHeight=iPos(4)-iPos(2);
      | iCx=iWidth/2;
      | iCy=iHeight/2;
      | [logoX, logoY] = xlogo(iPos);
      | [memX,memY] = memplot(iPos,min(depth,floor(iWidth/4)));
      | 
      | dataBPNum = 1;
      | dataBStr = '';
      | weBPNum = 1;
      | weBStr = '';
      | rstAPNum = 1;
      | rstAStr = '';
      | rstBPNum = 1;
      | rstBStr = '';
      | if(distributed_mem==0)
      |    dataBPNum = 5;
      |    dataBStr = 'data_B';
      |    weBPNum = 6;
      |    weBStr = 'we_B';
      |    if (latency==1)
      | 	   if (rst_a)
      | 		   rstAPNum = 7;
      | 		   rstAStr = 'rst_A';
      | 		   if (rst_b)
      | 	   			rstBPNum = 8;
      | 				rstBStr = 'rst_B';
      | 			end
      | 		else
      | 			if (rst_b)
      | 	   			rstBPNum = 7;
      | 				rstBStr = 'rst_B';
      | 			end
      | 		end
      |    end
      | end
      | 
      | voutAPNum = 1;
      | voutAStr = '';
      | voutBPNum = 1;
      | voutBStr = '';
      | doutBPNum=2;
      | if((mem_collision==1) && (distributed_mem==0) )
      |    voutAPNum = 2;
      |    voutAStr = 'vout_A';
      |    doutBPNum=3;
      |    voutBPNum = 4;
      |    voutBStr = 'vout_B';
      | end
      | 
      | % one time added for param list
      | useCore = 1;
      | dblOvrd = dbl_ovrd;
      | precision0 = 1;
      | precision1 = 1;
      | precision2 = 1;
      | precision3 = 1;
      | depthA = depth;
      | init = initVector;
      | write_mode_a = write_mode_A;
      | write_mode_b = write_mode_B;
      | initZero = init_zero;
      | explicitClk = explicit_period;
      | gen_core = 1;
      | 
      | % just pass everything to s-function
      | sfcn_mwsv__ = get_param(gcb, 'MaskWSVariables');
      mask Help: eval('xlWeb(xlhtmldoclink(''Dual Port RAM''))');
      mask StyleString: edit,edit,popup(Read After Write|Read Before Write|No Read On Write),popup(Read After Write|Read Before Write|No Read On Write),edit,checkbox,checkbox,checkbox,edit,checkbox,checkbox,edit,checkbox,edit,checkbox,checkbox,checkbox,checkbox,edit,checkbox
      mask CallbackString: |||||||xldpramCallback|||xldpramCallback||xldpramCallback||xldpramCallback|xldpramCallback||||
      mask Display:
      | patch([0 iWidth iWidth 0],[0 0 iHeight iHeight] ,bg);
      | patch([0 iWidth iWidth 0],[iCy-2 iCy-2 iCy+2 iCy+2] , .9* bg);
      | patch(logoX,logoY , fg);
      | port_label('input',1,'addr_A');
      | port_label('input',2,'data_A');
      | port_label('input',3,'we_A');
      | port_label('input',4,'addr_B');
      | port_label('input',dataBPNum,dataBStr);
      | port_label('input',weBPNum,weBStr);
      | port_label('input',rstAPNum,rstAStr);
      | port_label('input',rstBPNum,rstBStr);
      | port_label('output',1,'A');
      | port_label('output',doutBPNum,'B');
      | port_label('output',voutAPNum,voutAStr);
      | port_label('output',voutBPNum,voutBStr);
      | ;plot([0 0 iWidth iWidth 0], [0 iHeight iHeight 0 0]);
  wr_addr : xbsIndex_r3/Counter  cnt_type=Free Running  n_bits=11  bin_pt=0  arith_type=Unsigned  start_count=0  cnt_to=Inf  cnt_by_val=1  operation=Up  explicit_period=off  period=1  load_pin=off  rst=off  en=off  dbl_ovrd=off  show_param=off  use_rpm=on  gen_core=off
      settings: xl_area=[0, 0, 0, 0, 0, 0, 0]
  dout : Outport
  wires:
  Dual Port RAM/2 -> dout/1
  AddSub/1 -> Dual Port RAM/4
  delay/1 -> AddSub/2
  Constant4/1 -> Dual Port RAM/6
  din/1 -> Dual Port RAM/2, Dual Port RAM/5
  Constant2/1 -> Dual Port RAM/3
  wr_addr/1 -> Dual Port RAM/1, AddSub/1

== system poco_ref_al_r307/delay_wideband_prog0/delay_dp1 ==
  din : Inport  Port=1  LatchInput=off
  delay : Inport  Port=2  LatchInput=off
  AddSub : xbsIndex_r3/AddSub  mode=Subtraction  precision=User Defined  arith_type=Unsigned  n_bits=11  bin_pt=0  quantization=Truncate  overflow=Wrap  latency=1  explicit_period=off  period=1  use_carryin=off  use_carryout=off  en=off  dbl_ovrd=off  show_param=off  use_core=on  pipeline=off  use_rpm=on  gen_core=off
      settings: xl_area=[0, 0, 0, 0, 0, 0, 0]
  Constant2 : xbsIndex_r3/Constant  const=1  equ=P=C  arith_type=Boolean  n_bits=1  bin_pt=0  opselect=C  inp2=PCIN>>17  opr=+  inp1=P  carry=CIN  iostate=0  explicit_period=on  period=1  dbl_ovrd=off
  Constant4 : xbsIndex_r3/Constant  const=0  equ=P=C  arith_type=Boolean  n_bits=1  bin_pt=0  opselect=C  inp2=PCIN>>17  opr=+  inp1=P  carry=CIN  iostate=0  explicit_period=on  period=1  dbl_ovrd=off
  Dual Port RAM : S-Function  AncestorBlock=xbsIndex_r3/Dual Port RAM  FunctionName=xldpram  Parameters=sfcn_mwsv__  mask(Xilinx Dual Port Random Access Memory){depth=2048, initVector=0, write_mode_A=Read After Write, write_mode_B=Read After Write, latency=4, mem_collision=off, init_zero=on, explicit_period=off, period=1, dbl_ovrd=off, rst_a=off, init_a=0, rst_b=off, init_b=0, show_param=off, distributed_mem=off, use_rpm=off, gen_core=off, xl_area=[0, 0, 0, 0, 0, 0, 0], xl_use_area=off}
      mask prompts: initVector "Initial Value Vector"; write_mode_A "Write Mode:  Port A"; write_mode_B "Write Mode:  Port B"; mem_collision "Provide Output Valid Port"; init_zero "Zero Initial Output  (otherwise NaN)"; explicit_period "Use Explicit Sample Period"; period "Sample Period  (use -1 to inherit first known input period)"; dbl_ovrd "Override with Doubles"; rst_a "Provide Reset Port for Port A Output Register"; init_a "Initial Value for Port A Output Register"; rst_b "Provide Reset Port for Port B Output Register"; init_b "Initial Value for Port B Output Register"; show_param "---------------------- Show Implementation Parameters -----------------------------------------------------------------------------------"; distributed_mem "Use Distributed Memory (instead of block RAM)"; use_rpm "Use Placement Information for Core"; gen_core "Generate Core"; xl_area "FPGA Area [Slices, FFs, BRAMs, LUTs, IOBs, Emb. Mults, TBUFs]"; xl_use_area "Use Area Above For Estimation"
      mask help: Dual port random access memory (RAM). Independent address, data and write enable ports allow shared access to a single memory space. Dual ports enable simultaneous access to the memory space at different sample rates using multiple data widths.
      mask init: same as poco_ref_al_r307/delay_wideband_prog0/delay_dp/Dual Port RAM
      mask Help: eval('xlWeb(xlhtmldoclink(''Dual Port RAM''))');
      mask StyleString: edit,edit,popup(Read After Write|Read Before Write|No Read On Write),popup(Read After Write|Read Before Write|No Read On Write),edit,checkbox,checkbox,checkbox,edit,checkbox,checkbox,edit,checkbox,edit,checkbox,checkbox,checkbox,checkbox,edit,checkbox
      mask CallbackString: |||||||xldpramCallback|||xldpramCallback||xldpramCallback||xldpramCallback|xldpramCallback||||
      mask Display:
      | patch([0 iWidth iWidth 0],[0 0 iHeight iHeight] ,bg);
      | patch([0 iWidth iWidth 0],[iCy-2 iCy-2 iCy+2 iCy+2] , .9* bg);
      | patch(logoX,logoY , fg);
      | port_label('input',1,'addr_A');
      | port_label('input',2,'data_A');
      | port_label('input',3,'we_A');
      | port_label('input',4,'addr_B');
      | port_label('input',dataBPNum,dataBStr);
      | port_label('input',weBPNum,weBStr);
      | port_label('input',rstAPNum,rstAStr);
      | port_label('input',rstBPNum,rstBStr);
      | port_label('output',1,'A');
      | port_label('output',doutBPNum,'B');
      | port_label('output',voutAPNum,voutAStr);
      | port_label('output',voutBPNum,voutBStr);
      | ;plot([0 0 iWidth iWidth 0], [0 iHeight iHeight 0 0]);
  wr_addr : xbsIndex_r3/Counter  cnt_type=Free Running  n_bits=11  bin_pt=0  arith_type=Unsigned  start_count=0  cnt_to=Inf  cnt_by_val=1  operation=Up  explicit_period=off  period=1  load_pin=off  rst=off  en=off  dbl_ovrd=off  show_param=off  use_rpm=on  gen_core=off
      settings: xl_area=[0, 0, 0, 0, 0, 0, 0]
  dout : Outport
  wires:
  wr_addr/1 -> AddSub/1, Dual Port RAM/1
  Constant2/1 -> Dual Port RAM/3
  din/1 -> Dual Port RAM/5, Dual Port RAM/2
  Constant4/1 -> Dual Port RAM/6
  delay/1 -> AddSub/2
  AddSub/1 -> Dual Port RAM/4
  Dual Port RAM/2 -> dout/1

== system poco_ref_al_r307/delay_wideband_prog0/delay_dp2 ==
  din : Inport  Port=1  LatchInput=off
  delay : Inport  Port=2  LatchInput=off
  AddSub : xbsIndex_r3/AddSub  mode=Subtraction  precision=User Defined  arith_type=Unsigned  n_bits=11  bin_pt=0  quantization=Truncate  overflow=Wrap  latency=1  explicit_period=off  period=1  use_carryin=off  use_carryout=off  en=off  dbl_ovrd=off  show_param=off  use_core=on  pipeline=off  use_rpm=on  gen_core=off
      settings: xl_area=[0, 0, 0, 0, 0, 0, 0]
  Constant2 : xbsIndex_r3/Constant  const=1  equ=P=C  arith_type=Boolean  n_bits=1  bin_pt=0  opselect=C  inp2=PCIN>>17  opr=+  inp1=P  carry=CIN  iostate=0  explicit_period=on  period=1  dbl_ovrd=off
  Constant4 : xbsIndex_r3/Constant  const=0  equ=P=C  arith_type=Boolean  n_bits=1  bin_pt=0  opselect=C  inp2=PCIN>>17  opr=+  inp1=P  carry=CIN  iostate=0  explicit_period=on  period=1  dbl_ovrd=off
  Dual Port RAM : S-Function  AncestorBlock=xbsIndex_r3/Dual Port RAM  FunctionName=xldpram  Parameters=sfcn_mwsv__  mask(Xilinx Dual Port Random Access Memory){depth=2048, initVector=0, write_mode_A=Read After Write, write_mode_B=Read After Write, latency=4, mem_collision=off, init_zero=on, explicit_period=off, period=1, dbl_ovrd=off, rst_a=off, init_a=0, rst_b=off, init_b=0, show_param=off, distributed_mem=off, use_rpm=off, gen_core=off, xl_area=[0, 0, 0, 0, 0, 0, 0], xl_use_area=off}
      mask prompts: initVector "Initial Value Vector"; write_mode_A "Write Mode:  Port A"; write_mode_B "Write Mode:  Port B"; mem_collision "Provide Output Valid Port"; init_zero "Zero Initial Output  (otherwise NaN)"; explicit_period "Use Explicit Sample Period"; period "Sample Period  (use -1 to inherit first known input period)"; dbl_ovrd "Override with Doubles"; rst_a "Provide Reset Port for Port A Output Register"; init_a "Initial Value for Port A Output Register"; rst_b "Provide Reset Port for Port B Output Register"; init_b "Initial Value for Port B Output Register"; show_param "---------------------- Show Implementation Parameters -----------------------------------------------------------------------------------"; distributed_mem "Use Distributed Memory (instead of block RAM)"; use_rpm "Use Placement Information for Core"; gen_core "Generate Core"; xl_area "FPGA Area [Slices, FFs, BRAMs, LUTs, IOBs, Emb. Mults, TBUFs]"; xl_use_area "Use Area Above For Estimation"
      mask help: Dual port random access memory (RAM). Independent address, data and write enable ports allow shared access to a single memory space. Dual ports enable simultaneous access to the memory space at different sample rates using multiple data widths.
      mask init: same as poco_ref_al_r307/delay_wideband_prog0/delay_dp/Dual Port RAM
      mask Help: eval('xlWeb(xlhtmldoclink(''Dual Port RAM''))');
      mask StyleString: edit,edit,popup(Read After Write|Read Before Write|No Read On Write),popup(Read After Write|Read Before Write|No Read On Write),edit,checkbox,checkbox,checkbox,edit,checkbox,checkbox,edit,checkbox,edit,checkbox,checkbox,checkbox,checkbox,edit,checkbox
      mask CallbackString: |||||||xldpramCallback|||xldpramCallback||xldpramCallback||xldpramCallback|xldpramCallback||||
      mask Display:
      | patch([0 iWidth iWidth 0],[0 0 iHeight iHeight] ,bg);
      | patch([0 iWidth iWidth 0],[iCy-2 iCy-2 iCy+2 iCy+2] , .9* bg);
      | patch(logoX,logoY , fg);
      | port_label('input',1,'addr_A');
      | port_label('input',2,'data_A');
      | port_label('input',3,'we_A');
      | port_label('input',4,'addr_B');
      | port_label('input',dataBPNum,dataBStr);
      | port_label('input',weBPNum,weBStr);
      | port_label('input',rstAPNum,rstAStr);
      | port_label('input',rstBPNum,rstBStr);
      | port_label('output',1,'A');
      | port_label('output',doutBPNum,'B');
      | port_label('output',voutAPNum,voutAStr);
      | port_label('output',voutBPNum,voutBStr);
      | ;plot([0 0 iWidth iWidth 0], [0 iHeight iHeight 0 0]);
  wr_addr : xbsIndex_r3/Counter  cnt_type=Free Running  n_bits=11  bin_pt=0  arith_type=Unsigned  start_count=0  cnt_to=Inf  cnt_by_val=1  operation=Up  explicit_period=off  period=1  load_pin=off  rst=off  en=off  dbl_ovrd=off  show_param=off  use_rpm=on  gen_core=off
      settings: xl_area=[0, 0, 0, 0, 0, 0, 0]
  dout : Outport
  wires:
  Dual Port RAM/2 -> dout/1
  AddSub/1 -> Dual Port RAM/4
  delay/1 -> AddSub/2
  Constant4/1 -> Dual Port RAM/6
  din/1 -> Dual Port RAM/2, Dual Port RAM/5
  Constant2/1 -> Dual Port RAM/3
  wr_addr/1 -> Dual Port RAM/1, AddSub/1
